simulink model "verify_thermal_conductivity_mdl"  (Simulink 7.6)
settings: Solver=FixedStepDiscrete  StartTime=0.0  StopTime=1  FixedStep=1  RelTol=1e-3
values from neighbouring files (symbols this model uses):
  fmix = mix(n)    [verification_density.m]    (also in verification_fluidproperty.m; verification_heat_capacity.m; verification_kinematic_viscosity.m; verification_thermal_conductivity.m)
  press = p(m)    [verification_density.m]    (also in verification_fluidproperty.m; verification_heat_capacity.m; verification_kinematic_viscosity.m; verification_thermal_conductivity.m)
undefined symbols (not defined in the file or in its folder): fluid
libraries: carnot x1
settings Model: Creator=drhf  LastModifiedBy=drhf
settings DataIOCC: SaveTime=off  ReturnWorkspaceOutputs=on  OutputSaveName=rho2

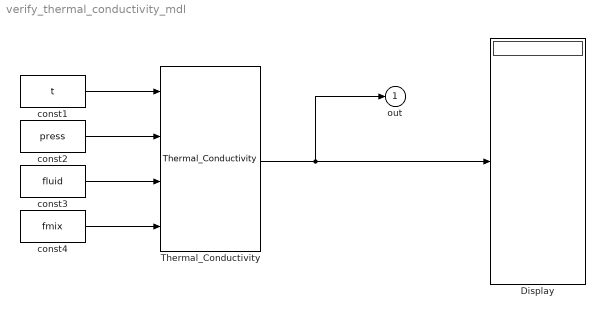
== system verify_thermal_conductivity_mdl ==
  Display : Display
  Thermal_Conductivity : carnot/Basic/Material_Properties/Thermal_Conductivity  SystemSampleTime=-1  VariantObject=CarlibClassic  INPUTARGUMENTS=state variables (classic)  DEBUGLEVEL=WARNINGLEVEL  MAXTOTALMESSAGES=0  MAXCONSECUTIVEMESSAGES=0  WRITETOFILE=0  FILENAME='errors.txt'
  const1 : Constant  Value=t
  const2 : Constant  Value=press
  const3 : Constant  Value=fluid
  const4 : Constant  Value=fmix
  out : Outport  InitialOutput=0
  wires:
  Thermal_Conductivity/1 -> Display/1, out/1
  const1/1 -> Thermal_Conductivity/1
  const2/1 -> Thermal_Conductivity/2
  const3/1 -> Thermal_Conductivity/3
  const4/1 -> Thermal_Conductivity/4
